simulink model "gemerapresim"  (R2023b)
settings: Solver=ode4  StartTime=0.0  StopTime=250  FixedStep=0.0001  RelTol=1e-3
undefined symbols (not defined in the file): Af, C0, C1, Cd, g, m, Rho, rwh
libraries: slpidlib x1
settings Model: Creator=saman  LastModifiedBy=saman

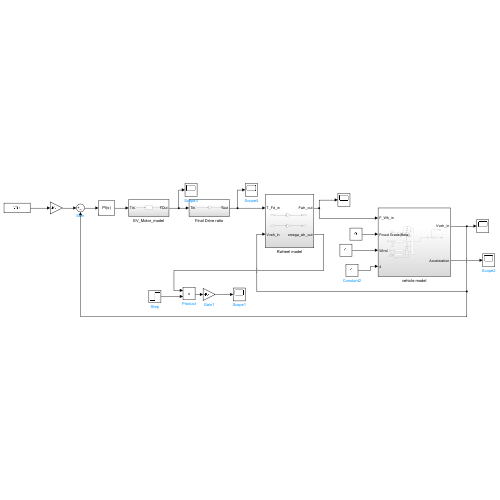
[thumbnail: Simulink's stored preview of the top-level diagram]
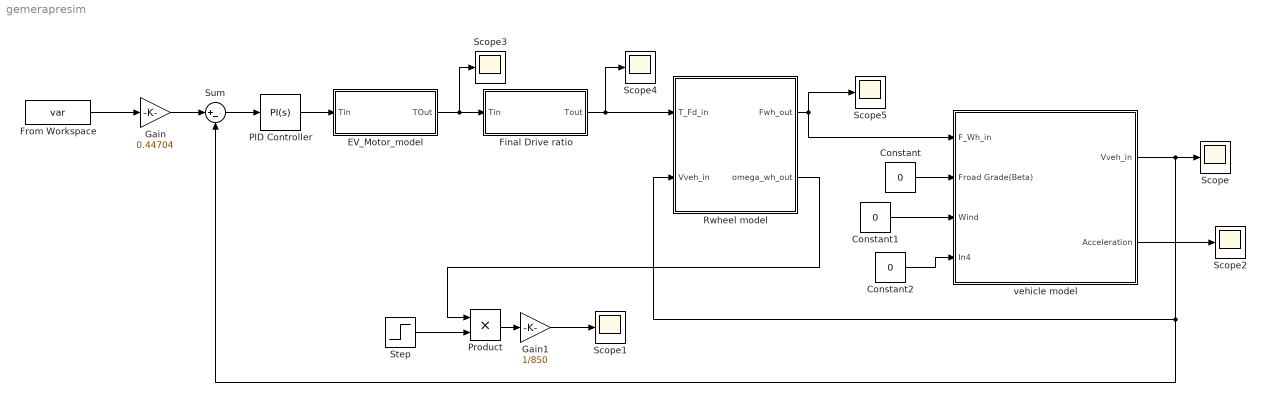
== system gemerapresim ==
  Constant : Constant  Value=0
  Constant1 : Constant  Value=0
  Constant2 : Constant  Value=0
  EV_Motor_model : Subsystem
  Final Drive ratio : Subsystem
  From Workspace : FromWorkspace  VariableName=var
  Gain : Gain  Gain=0.44704
  Gain1 : Gain  Gain=1/850
  PID Controller : slpidlib/PID Controller  Controller=PI  Form=Parallel  TimeDomain=Continuous-time  UseExternalTs=off  SampleTime=-1  IntegratorMethod=Forward Euler  FilterMethod=Forward Euler  ControllerParametersSource=internal  P=10000  I=5000  UseKiTs=off  D=0  N=100  UseFilter=on  TunerSelectOption=Transfer Function Based (PID Tuner App)  InitialConditionSource=internal  InitialConditionForIntegrator=0  InitialConditionForFilter=0  DifferentiatorICPrevScaledInput=0  ExternalReset=none  TrackingMode=off  Kt=1  LimitOutput=off  SatLimitsSource=internal  UpperSaturationLimit=inf  LowerSaturationLimit=-inf  LinearizeAsGain=on  AntiWindupMode=none  Kb=1  LimitIntegrator=off  UpperIntegratorSaturationLimit=inf  LowerIntegratorSaturationLimit=-inf  POutMin=[]  POutMax=[]  IOutMin=[]  IOutMax=[]  DOutMin=[]  DOutMax=[]  NOutMin=[]  NOutMax=[]  SumOutMin=[]  SumOutMax=[]  SaturationOutMin=[]  SaturationOutMax=[]  PParamMin=[]  PParamMax=[]  IParamMin=[]  IParamMax=[]  DParamMin=[]  DParamMax=[]  NParamMin=[]  NParamMax=[]  KbParamMin=[]  KbParamMax=[]  KtParamMin=[]  KtParamMax=[]  KbOutMin=[]  KbOutMax=[]  KtOutMin=[]  KtOutMax=[]  IntegratorOutMin=[]  IntegratorOutMax=[]  FilterOutMin=[]  FilterOutMax=[]  SumI1OutMin=[]  SumI1OutMax=[]  SumI2OutMin=[]  SumI2OutMax=[]  SumI3OutMin=[]  SumI3OutMax=[]  SumI4OutMin=[]  SumI4OutMax=[]  SumDOutMin=[]  SumDOutMax=[]  DifferentiatorOutMin=[]  DifferentiatorOutMax=[]  FilterDiffOutCoefMin=[]  FilterDiffOutCoefMax=[]  ReciprocalOutMin=[]  ReciprocalOutMax=[]  SumDenOutMin=[]  SumDenOutMax=[]  SumNumOutMin=[]  SumNumOutMax=[]  DivideOutMin=[]  DivideOutMax=[]  UdiffTsProdOutMin=[]  UdiffTsProdOutMax=[]  NTsProdOutMin=[]  NTsProdOutMax=[]  UintegralTsProdOutMin=[]  UintegralTsProdOutMax=[]  UngainTsProdOutMin=[]  UngainTsProdOutMax=[]  ClampingZeroOutDataTypeStr=Inherit: Inherit via back propagation  ClampingZeroOutMin=[]  ClampingZeroOutMax=[]  FilterDenConstantOutDataTypeStr=Inherit: Inherit via back propagation  FilterDenConstantOutMin=[]  FilterDenConstantOutMax=[]  PCopyOutDataTypeStr=Inherit: Inherit via back propagation  PCopyOutMin=[]  PCopyOutMax=[]  NCopyOutDataTypeStr=Inherit: Inherit via back propagation  NCopyOutMin=[]  NCopyOutMax=[]  IntegratorContinuousStateAttributes=''  IntegratorStateMustResolveToSignalObject=off  IntegratorRTWStateStorageClass=Auto  FilterContinuousStateAttributes=''  FilterStateMustResolveToSignalObject=off  FilterRTWStateStorageClass=Auto  ParallelPVariant=InternalParameters  IdealPVariant=Disabled  IVariant=InternalParameters  DVariant=Disabled  IntegratorVariant=Continuous  SatVariant=Disabled  AWVariant=Passthrough  PCopyVariant=Disabled  TRVariant=Disabled  FdbkBlocksVariant=Forward  IdealPFdbkVariant=Disabled  SatFdbkVariant=Disabled  DerivativeFilterVariant=Disabled  NVariant=Disabled  NCopyVariant=Disabled_SignalSpec  FilterICVariant=Disabled  IntegratorICVariant=InternalICs  ExternalResetVariant=Disabled  TRSumVariant=Passthrough  SumFdbkVariant=Disabled  SumVariant=Sum_PI  TsampFilterVariant=InternalTs  TsampNgainVariant=Passthrough  TsampIntegralVariant=Disabled_SignalSpec  ExternalSaturationOutDataTypeStr=Inherit: Same as second input
  Product : Product
  Rwheel model : Subsystem
  Scope{,1..5} (6 alike) : Scope
  Step : Step  After=600  SampleTime=0
  Sum : Sum  Inputs=|+-
  vehicle model : Subsystem
  wires:
  vehicle model/1(Vveh_in) -> Sum/2, Rwheel model/2(Vveh_in), Scope/1
  Rwheel model/1(Fwh_out) -> Scope5/1, vehicle model/1(F_Wh_in)
  EV_Motor_model/1(TOut) -> Scope3/1, Final Drive ratio/1(Tin)
  Constant1/1 -> vehicle model/3(Wind)
  Constant/1 -> vehicle model/2(Froad Grade(Beta))
  vehicle model/2(Acceleration) -> Scope2/1
  Constant2/1 -> vehicle model/4(In4)
  Final Drive ratio/1(Tout) -> Scope4/1, Rwheel model/1(T_Fd_in)
  PID Controller/1 -> EV_Motor_model/1(Tin)
  Sum/1 -> PID Controller/1
  Gain/1 -> Sum/1
  From Workspace/1 -> Gain/1
  Rwheel model/2(omega_wh_out) -> Product/1
  Step/1 -> Product/2
  Product/1 -> Gain1/1
  Gain1/1 -> Scope1/1

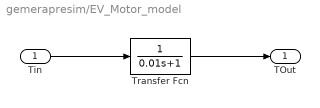
== system gemerapresim/EV_Motor_model ==
  Tin : Inport
  Transfer Fcn : TransferFcn  Denominator=[0.01 1]
  TOut : Outport
  wires:
  Tin/1 -> Transfer Fcn/1
  Transfer Fcn/1 -> TOut/1

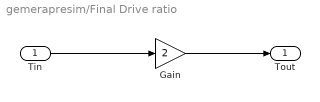
== system gemerapresim/Final Drive ratio ==
  Tin : Inport
  Gain : Gain  Gain=2
  Tout : Outport
  wires:
  Tin/1 -> Gain/1
  Gain/1 -> Tout/1

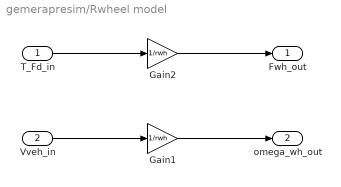
== system gemerapresim/Rwheel model ==
  T_Fd_in : Inport
  Vveh_in : Inport  Port=2
  Gain1 : Gain  Gain=1/rwh
  Gain2 : Gain  Gain=1/rwh
  Fwh_out : Outport
  omega_wh_out : Outport  Port=2
  wires:
  T_Fd_in/1 -> Gain2/1
  Vveh_in/1 -> Gain1/1
  Gain1/1 -> omega_wh_out/1
  Gain2/1 -> Fwh_out/1

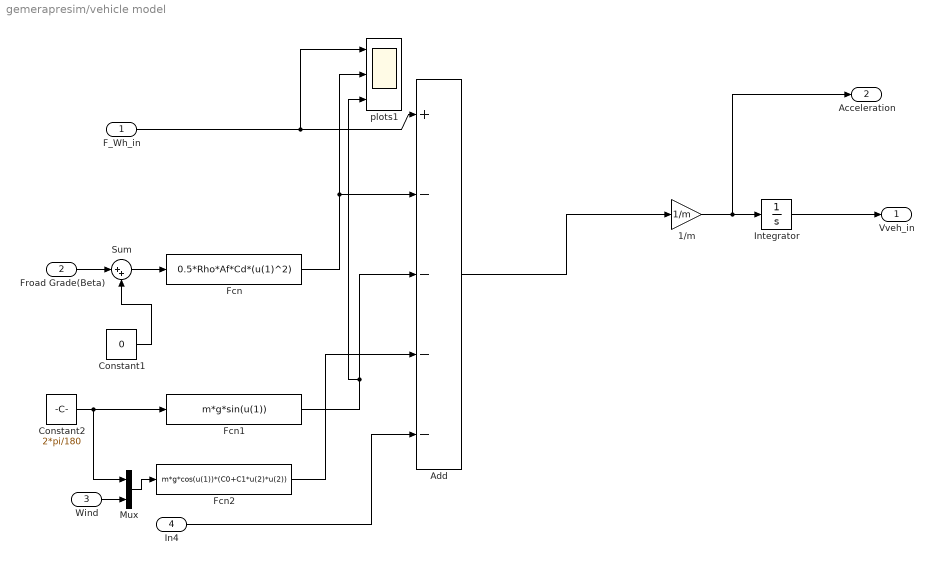
== system gemerapresim/vehicle model ==
  F_Wh_in : Inport
  Froad Grade(Beta) : Inport  Port=2
  Wind : Inport  Port=3
  In4 : Inport  Port=4
  1/m : Gain  Gain=1/m
  Add : Sum  Inputs=+----
  Constant1 : Constant  Value=0
  Constant2 : Constant  Value=2*pi/180
  Fcn : Fcn  Expr=0.5*Rho*Af*Cd*(u(1)^2)
  Fcn1 : Fcn  Expr=m*g*sin(u(1))
  Fcn2 : Fcn  Expr=m*g*cos(u(1))*(C0+C1*u(2)*u(2))
  Integrator : Integrator
  Mux : Mux  Inputs=2
  Sum : Sum  Inputs=|++
  plots1 : Scope  NumInputPorts=3
  Vveh_in : Outport
  Acceleration : Outport  Port=2
  wires:
  Fcn/1 -> plots1/2, Add/2
  Add/1 -> 1/m/1
  1/m/1 -> Acceleration/1, Integrator/1
  Fcn1/1 -> plots1/3, Add/3
  Integrator/1 -> Vveh_in/1
  F_Wh_in/1 -> plots1/1, Add/1
  Sum/1 -> Fcn/1
  Froad Grade(Beta)/1 -> Sum/1
  Constant1/1 -> Sum/2
  Fcn2/1 -> Add/4
  Wind/1 -> Mux/2
  Constant2/1 -> Mux/1, Fcn1/1
  Mux/1 -> Fcn2/1
  In4/1 -> Add/5
